simulink model "qcar2LidarToGPS"  (R2023a)
settings: Solver=ode1  StartTime=0.0  StopTime=inf  FixedStep=1/15  RelTol=1e-3  EnableMultiTasking=on
undefined symbols (not defined in the file): Point, qc_get_step_size
libraries: quarc_library x20, simulink x4
settings Model: SimulationMode=external  ExtModeTrigDuration=10000  Creator=PKaram  LastModifiedBy=ZinanCen
settings SolverCC: AlgebraicLoopSolver=TrustRegion  PositivePriorityOrder=on  AutoInsertRateTranBlk=on
settings DataIOCC: ReturnWorkspaceOutputs=off
settings DebuggingCC: ParameterPrecisionLossMsg=none  UnconnectedInputMsg=warning  UnconnectedOutputMsg=warning  UnconnectedLineMsg=warning  ArithmeticOperatorsInVariantConditions=warning
settings HardwareCC: ProdBitPerLong=64  ProdLargestAtomicInteger=LongLong  ProdLargestAtomicFloat=Double  ProdLongLongMode=on  ProdHWDeviceType=ARM Compatible->ARM 64-bit (LP64)
settings ModelReferenceCC: EnableRefExpFcnMdlSchedulingChecks=on
settings SFSimCC: SimUseLocalCustomCode=off  CustomCodeUndefinedFunction=UseInterfaceOnly
settings RTWCC: Description=QUARC Linux QCar2 Target Using Toolchain  SystemTargetFile=quarc_linux_qcar2.tlc  TemplateMakefile=quarc_linux_nvidia_tmf  RTWUseLocalCustomCode=off  Toolchain=QUARC linux_qcar2 | gmake (64-bit Windows)  BuildConfiguration=Faster Runs  DLArmComputeVersion=19.05
settings CodeAppCC: StateflowObjectComments=on
settings STFCustomTargetCC: SystemTargetFile=quarc_linux_qcar2.tlc
settings GRTTargetCC: ParMdlRefBuildCompliant=off  CompOptLevelCompliant=off  CombineOutputUpdateFcns=off  MatFileLogging=off  CPPClassGenCompliant=off  GRTInterface=on  ExtMode=on  ExtModeMexFile=quarc_comm  ExtModeMexArgs='-w -d /home/nvidia/Documents -uri %u -pose_0 [0.],[0.],[0.]','tcpip://192.168.3.38:17001'
settings ConfigComp: CovMetricSettings=dswe

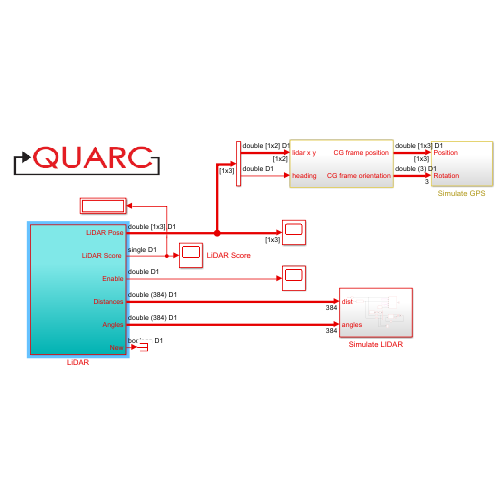
[thumbnail: Simulink's stored preview of the top-level diagram]
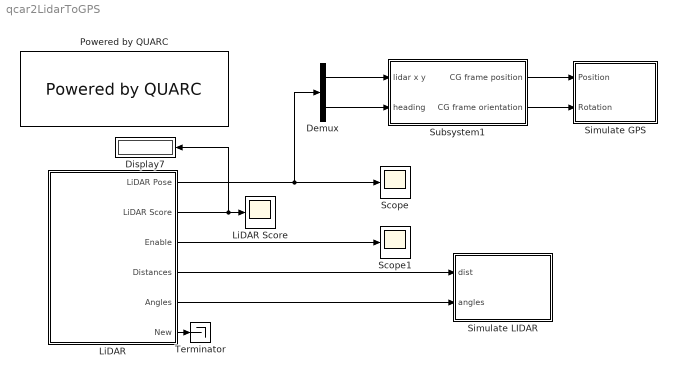
== system qcar2LidarToGPS ==
  Demux : Demux  Outputs=[2 1]
  Display7 : Display
  LiDAR : Subsystem
  LiDAR Score : Scope
  Powered by QUARC : quarc_library/Logos/Powered by QUARC
  Scope : Scope
  Scope1 : Scope
  Simulate GPS : Subsystem
  Simulate LIDAR : Subsystem
  Subsystem1 : Subsystem
  Terminator : Terminator
  wires:
  LiDAR/2("LiDAR Score ") -> Display7/1, LiDAR Score/1
  LiDAR/3(Enable) -> Scope1/1
  LiDAR/1(LiDAR Pose) -> Scope/1, Demux/1
  Demux/1 -> Subsystem1/1(lidar x y)
  Subsystem1/1("CG frame position ") -> Simulate GPS/1(Position)
  Subsystem1/2(CG frame orientation) -> Simulate GPS/2(Rotation)
  Demux/2 -> Subsystem1/2(heading)
  LiDAR/4(Distances) -> Simulate LIDAR/1(dist)
  LiDAR/5(Angles) -> Simulate LIDAR/2(angles)
  LiDAR/6(New) -> Terminator/1

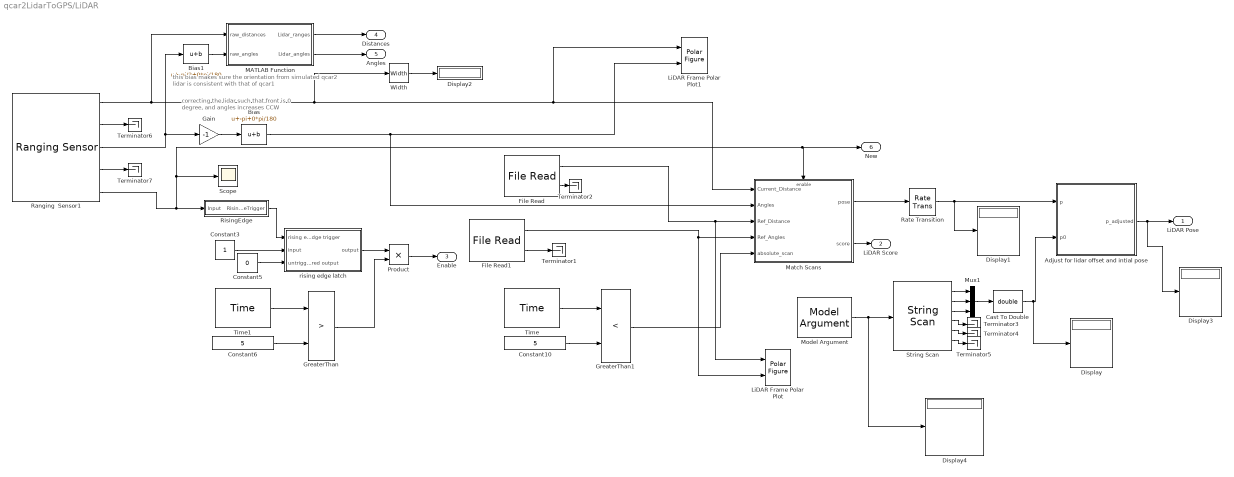
== system qcar2LidarToGPS/LiDAR ==
  note: correcting the lidar such that front is 0 degree, and angles increases CCW
  note: this bias makes sure the orientation from simulated qcar2 lidar is consistent with that of qcar1
  Adjust for lidar offset and intial pose : MATLAB Function  TreatAsAtomicUnit=on
  Bias : Bias  Bias=-pi+0*pi/180  SaturateOnIntegerOverflow=off
  Bias1 : Bias  Bias=-pi/2+0*pi/180  SaturateOnIntegerOverflow=off
  Cast To Double : DataTypeConversion  OutDataTypeStr=double  SaturateOnIntegerOverflow=off  RndMeth=Floor
  Constant10 : Constant  Value=5
  Constant3 : Constant
  Constant5 : Constant  Value=0
  Constant6 : Constant  Value=5
  Display{,1..4} (5 alike) : Display
  File Read : quarc_library/Sources/Signals/File Read  source=Specify via dialog (do not evaluate)  filename=distance_new.mat  format=MAT-file v.4  variable=distances  dimensions=[384, 1]  skip_lines=1  skip_columns=1  loop_count=0  sample_time=qc_get_step_size  data_type=double
      settings: AttributesFormatString="\"distance_new.mat"  SourceProductName=QUARC Targets
  File Read1 : quarc_library/Sources/Signals/File Read  source=Specify via dialog (do not evaluate)  filename=angles_new.mat  format=MAT-file v.4  variable=angles  dimensions=[384, 1]  skip_lines=1  skip_columns=1  loop_count=0  sample_time=qc_get_step_size  data_type=double
      settings: AttributesFormatString="\"angles_new.mat"  SourceProductName=QUARC Targets
  Gain : Gain  Gain=-1
  GreaterThan : RelationalOperator  Operator=>  OutDataTypeStr=boolean  RndMeth=Simplest  InputSameDT=off
  GreaterThan1 : RelationalOperator  Operator=<  OutDataTypeStr=boolean  RndMeth=Simplest  InputSameDT=off
  LiDAR Frame Polar Plot : quarc_library/Sinks/Figures/Polar Figure  figure_mode=Use figure window  figure_tag=figure1  axes_tag=axes1  plot_mode=Frame-based  minimum_rho=0  maximum_rho=5  minimum_theta=0  maximum_theta=360  zero_location=top  direction=counterclockwise  buffer_size=1  update_rate=1  sample_time=-1  initial_position="1541.8           49.8          766.4          758.4"  initial_visibility=off  line1_style=None  line1_width=1  line1_color=[0 0 0]  marker1=Point (.)  marker1_size=1  marker1_edge_color=[0 0.447059 0.741176]  marker1_face_color=[0 0.447059 0.741176]  line2_style=Solid line (-)  line2_width=0.5  line2_color=[0.85098 0.32549 0.0980392]  marker2=None  marker2_size=6  marker2_edge_color=[0.85098 0.32549 0.0980392]  marker2_face_color=[0.85098 0.32549 0.0980392]  line3_style=Solid line (-)  line3_width=0.5  line3_color=[0.929412 0.694118 0.12549]  marker3=None  marker3_size=6  marker3_edge_color=[0.929412 0.694118 0.12549]  marker3_face_color=[0.929412 0.694118 0.12549]  line4_style=Solid line (-)  line4_width=0.5  line4_color=[0.494118 0.184314 0.556863]  marker4=None  marker4_size=6  marker4_edge_color=[0.494118 0.184314 0.556863]  marker4_face_color=[0.494118 0.184314 0.556863]  line5_style=Solid line (-)  line5_width=0.5  line5_color=[0.466667 0.67451 0.188235]  marker5=None  marker5_size=6  marker5_edge_color=[0.466667 0.67451 0.188235]  marker5_face_color=[0.466667 0.67451 0.188235]
      settings: SourceProductName=QUARC Targets
  LiDAR Frame Polar Plot1 : quarc_library/Sinks/Figures/Polar Figure  figure_mode=Use figure window  figure_tag=figure1  axes_tag=axes1  plot_mode=Frame-based  minimum_rho=0  maximum_rho=5  minimum_theta=0  maximum_theta=360  zero_location=top  direction=counterclockwise  buffer_size=1  update_rate=1  sample_time=-1  initial_position="2305.8           49.8          766.4          758.4"  initial_visibility=off  line1_style=None  line1_width=1  line1_color=[0 0 0]  marker1=Point (.)  marker1_size=1  marker1_edge_color=[0 0.447059 0.741176]  marker1_face_color=[0 0.447059 0.741176]  line2_style=Solid line (-)  line2_width=0.5  line2_color=[0.85098 0.32549 0.0980392]  marker2=None  marker2_size=6  marker2_edge_color=[0.85098 0.32549 0.0980392]  marker2_face_color=[0.85098 0.32549 0.0980392]  line3_style=Solid line (-)  line3_width=0.5  line3_color=[0.929412 0.694118 0.12549]  marker3=None  marker3_size=6  marker3_edge_color=[0.929412 0.694118 0.12549]  marker3_face_color=[0.929412 0.694118 0.12549]  line4_style=Solid line (-)  line4_width=0.5  line4_color=[0.494118 0.184314 0.556863]  marker4=None  marker4_size=6  marker4_edge_color=[0.494118 0.184314 0.556863]  marker4_face_color=[0.494118 0.184314 0.556863]  line5_style=Solid line (-)  line5_width=0.5  line5_color=[0.466667 0.67451 0.188235]  marker5=None  marker5_size=6  marker5_edge_color=[0.466667 0.67451 0.188235]  marker5_face_color=[0.466667 0.67451 0.188235]
      settings: SourceProductName=QUARC Targets
  MATLAB Function : MATLAB Function  TreatAsAtomicUnit=on
  Match Scans : Subsystem
  Model Argument : quarc_library/Sources/Signals/Model Argument  argument_name=pose_0  has_value=on  data_type_mode=Specify via dialog  data_type=char  max_length=80  default_value=0  default_string=0,0,0  variable_size=on
      settings: AttributesFormatString=(-%<argument_name>)  SourceProductName=QUARC Targets
  Mux1 : Mux  Inputs=3
  Product : Product
  Ranging  Sensor1 : quarc_library/Devices/Third-Party/Sensors/Ranging Sensor  sensor_type=RPLidar LIDAR  uri=serial-cpu://localhost:1?baud='256000',word='8',parity='none',stop='1',flow='none',dsr='on'  ranging_distance=Long  timing_budget=0.033  measurement_period=0.0005  output_mode=Fixed-size interpolated output  samples_per_revolution=384  max_distance=0.050  max_angle=5  sample_time=qc_get_step_size  show_versions=off  active=on
      settings: SourceProductName=QUARC Targets
  Rate Transition : RateTransition
  RisingEdge : Subsystem
  Scope : Scope
  String Scan : quarc_library/Strings/String Scan  format_string=%e, %f, %g  max_length=80
      settings: SourceProductName=QUARC Targets
  Terminator{1..7} (7 alike) : Terminator
  Time : quarc_library/Sources/Time/Time  time_source=Wall clock  sample_time=qc_get_step_size
  Time1 : quarc_library/Sources/Time/Time  time_source=Wall clock  sample_time=qc_get_step_size
  Width : Width
  rising edge latch : Subsystem
  LiDAR Pose : Outport
  "LiDAR Score " : Outport  Port=2
  Enable : Outport  Port=3
  Distances : Outport  Port=4
  Angles : Outport  Port=5
  New : Outport  Port=6
  wires:
  File Read/1 -> LiDAR Frame Polar Plot/1, Match Scans/3(Ref_Distance)
  Width/1 -> Display2/1
  Ranging  Sensor1/1 -> MATLAB Function/1(raw_distances), Width/1, LiDAR Frame Polar Plot1/1, Match Scans/1(Current_Distance)
  Match Scans/1(pose) -> Rate Transition/1
  Constant6/1 -> GreaterThan/2
  RisingEdge/1(RisingEdgeTrigger) -> rising edge latch/1(rising edge trigger)
  Match Scans/2(score) -> "LiDAR Score "/1
  Product/1 -> Enable/1
  Constant3/1 -> rising edge latch/2(input)
  Constant5/1 -> rising edge latch/3(untriggered output)
  Constant10/1 -> GreaterThan1/2
  GreaterThan/1 -> Product/2
  Time/1 -> GreaterThan1/1
  GreaterThan1/1 -> Match Scans/5(absolute_scan)
  Time1/1 -> GreaterThan/1
  rising edge latch/1(output) -> Product/1
  Bias/1 -> Match Scans/2(Angles), LiDAR Frame Polar Plot1/2
  Ranging  Sensor1/5 -> New/1, Match Scans/Enable, Scope/1, RisingEdge/1(Input)
  File Read1/1 -> LiDAR Frame Polar Plot/2, Match Scans/4(Ref_Angles)
  File Read1/2 -> Terminator1/1
  File Read/2 -> Terminator2/1
  Model Argument/1 -> Display4/1, String Scan/1
  String Scan/4 -> Terminator3/1
  String Scan/5 -> Terminator4/1
  String Scan/6 -> Terminator5/1
  MATLAB Function/1(Lidar_ranges) -> Distances/1
  MATLAB Function/2(Lidar_angles) -> Angles/1
  Mux1/1 -> Cast To Double/1
  String Scan/1 -> Mux1/1
  String Scan/2 -> Mux1/2
  String Scan/3 -> Mux1/3
  Adjust for lidar offset and intial pose/1(p_adjusted) -> Display3/1, LiDAR Pose/1
  Rate Transition/1 -> Display1/1, Adjust for lidar offset and intial pose/1(p)
  Cast To Double/1 -> Display/1, Adjust for lidar offset and intial pose/2(p0)
  Ranging  Sensor1/2 -> Terminator6/1
  Ranging  Sensor1/4 -> Terminator7/1
  Gain/1 -> Bias/1
  Ranging  Sensor1/3 -> Bias1/1, Gain/1
  Bias1/1 -> MATLAB Function/2(raw_angles)

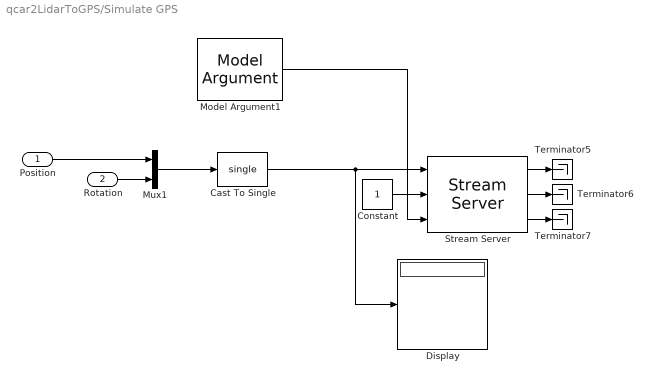
== system qcar2LidarToGPS/Simulate GPS ==
  Position : Inport
  Rotation : Inport  Port=2
  Cast To Single : DataTypeConversion  OutDataTypeStr=single  SaturateOnIntegerOverflow=off  RndMeth=Floor
  Constant : Constant
  Display : Display
  Model Argument1 : quarc_library/Sources/Signals/Model Argument  argument_name=uri_gps  has_value=on  data_type_mode=Specify via dialog  data_type=char  max_length=80  default_value=0  default_string=tcpip://remotehost:18967  variable_size=off
      settings: AttributesFormatString=(-%<argument_name>)  SourceProductName=QUARC Targets
  Mux1 : Mux  Inputs=2
  Stream Server : quarc_library/Communications/Basic/Stream Server  uri_source=External input port  uri=tcpip://remotehost:18967  send_buffer_size=1460  receive_buffer_size=1460  byte_order=little endian (Intel - LSB first)  optimization=Minimum latency  send_options=Send most recent data  receive_options=Do not receive data  default_value=[0]  sample_time=qc_get_step_size*3  active=off  implementation=Use blocking I/O in a separate thread  send_fifo_size=1000  receive_fifo_size=1000  send_priority=0  receive_priority=0  send_dimensions=off  receive_dimensions=off  max_dimensions=-1  data_type=Inherited via back propagation  type_expr=BusObject
  Terminator5 : Terminator
  Terminator6 : Terminator
  Terminator7 : Terminator
  wires:
  Rotation/1 -> Mux1/2
  Stream Server/1 -> Terminator5/1
  Stream Server/2 -> Terminator6/1
  Stream Server/3 -> Terminator7/1
  Constant/1 -> Stream Server/2
  Position/1 -> Mux1/1
  Mux1/1 -> Cast To Single/1
  Cast To Single/1 -> Display/1, Stream Server/1
  Model Argument1/1 -> Stream Server/3

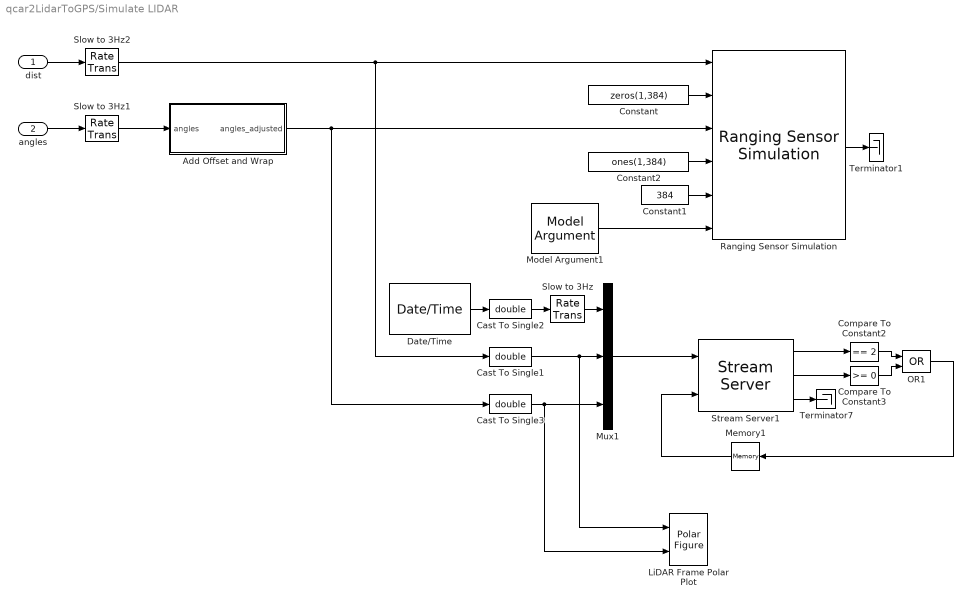
== system qcar2LidarToGPS/Simulate LIDAR ==
  dist : Inport
  angles : Inport  Port=2
  Add Offset and Wrap : MATLAB Function  TreatAsAtomicUnit=on
  Cast To Single1 : DataTypeConversion  OutDataTypeStr=double  SaturateOnIntegerOverflow=off  RndMeth=Floor
  Cast To Single2 : DataTypeConversion  OutDataTypeStr=double  SaturateOnIntegerOverflow=off  RndMeth=Floor
  Cast To Single3 : DataTypeConversion  OutDataTypeStr=double  SaturateOnIntegerOverflow=off  RndMeth=Floor
  Compare To Constant2 : simulink/Logic and Bit Operations/Compare To Constant  relop===  const=2  OutDataTypeStr=boolean
  Compare To Constant3 : simulink/Logic and Bit Operations/Compare To Constant  relop=>=  const=0  OutDataTypeStr=boolean
  Constant : Constant  Value=zeros(1,384)
  Constant1 : Constant  Value=384
  Constant2 : Constant  Value=ones(1,384)
  Date/Time : quarc_library/Sources/Time/Date//Time  show_date=off  show_time=off  show_epoch=on  use_utc=off  sample_time=-1
      settings: SourceProductName=QUARC Targets
  LiDAR Frame Polar Plot : quarc_library/Sinks/Figures/Polar Figure  figure_mode=Use figure window  figure_tag=figure1  axes_tag=axes1  plot_mode=Frame-based  minimum_rho=0  maximum_rho=5  minimum_theta=0  maximum_theta=360  zero_location=top  direction=counterclockwise  buffer_size=1  update_rate=1  sample_time=-1  initial_position="2306.3333      50.333333      765.33333      758.66667"  initial_visibility=off  line1_style=None  line1_width=1  line1_color=[0 0 0]  marker1=Point (.)  marker1_size=1  marker1_edge_color=[0 0.447059 0.741176]  marker1_face_color=[0 0.447059 0.741176]  line2_style=Solid line (-)  line2_width=0.5  line2_color=[0.85098 0.32549 0.0980392]  marker2=None  marker2_size=6  marker2_edge_color=[0.85098 0.32549 0.0980392]  marker2_face_color=[0.85098 0.32549 0.0980392]  line3_style=Solid line (-)  line3_width=0.5  line3_color=[0.929412 0.694118 0.12549]  marker3=None  marker3_size=6  marker3_edge_color=[0.929412 0.694118 0.12549]  marker3_face_color=[0.929412 0.694118 0.12549]  line4_style=Solid line (-)  line4_width=0.5  line4_color=[0.494118 0.184314 0.556863]  marker4=None  marker4_size=6  marker4_edge_color=[0.494118 0.184314 0.556863]  marker4_face_color=[0.494118 0.184314 0.556863]  line5_style=Solid line (-)  line5_width=0.5  line5_color=[0.466667 0.67451 0.188235]  marker5=None  marker5_size=6  marker5_edge_color=[0.466667 0.67451 0.188235]  marker5_face_color=[0.466667 0.67451 0.188235]
      settings: SourceProductName=QUARC Targets
  Memory1 : Memory  InheritSampleTime=on
  Model Argument1 : quarc_library/Sources/Signals/Model Argument  argument_name=uri_lidar  has_value=on  data_type_mode=Specify via dialog  data_type=char  max_length=80  default_value=0  default_string=tcpip://localhost:18966  variable_size=off
      settings: AttributesFormatString=(-%<argument_name>)  SourceProductName=QUARC Targets
  Mux1 : Mux  Inputs=3
  OR1 : Logic  Operator=OR  IconShape=distinctive  AllPortsSameDT=off  OutDataTypeStr=boolean
  Ranging Sensor Simulation : quarc_library/Devices/Third-Party/Sensors/Ranging Sensor Simulation  sensor_type=RPLIDAR A2  uri_source=External input port  uri=tcpip://localhost:18966  sample_time=qc_get_step_size  show_in_use=off  variable_size=off  active=on
      settings: SourceProductName=QUARC Targets
  Slow to 3Hz : RateTransition  OutPortSampleTime=qc_get_step_size*ceil(1/15 / qc_get_step_size)
  Slow to 3Hz1 : RateTransition  OutPortSampleTime=qc_get_step_size*ceil(1/15 / qc_get_step_size)
  Slow to 3Hz2 : RateTransition  OutPortSampleTime=qc_get_step_size*ceil(1/15 / qc_get_step_size)
  Stream Server1 : quarc_library/Communications/Basic/Stream Server  uri_source=Specify via dialog (do not evaluate)  uri=tcpip://localhost:18968  send_buffer_size=8*(384*2 +1)  receive_buffer_size=1  byte_order=little endian (Intel - LSB first)  optimization=Minimum latency  send_options=Send most recent data  receive_options=Do not receive data  default_value=[0]  sample_time=qc_get_step_size*ceil(1/15 / qc_get_step_size)  active=off  implementation=Use non-blocking I/O  send_fifo_size=1  receive_fifo_size=1000  send_priority=0  receive_priority=0  send_dimensions=off  receive_dimensions=off  max_dimensions=-1  data_type=Inherited via back propagation  type_expr=BusObject
      settings: AttributesFormatString="\"tcpip://localhost:18968\""
  Terminator1 : Terminator
  Terminator7 : Terminator
  wires:
  Constant/1 -> Ranging Sensor Simulation/2
  Constant1/1 -> Ranging Sensor Simulation/5
  Constant2/1 -> Ranging Sensor Simulation/4
  Ranging Sensor Simulation/1 -> Terminator1/1
  dist/1 -> Slow to 3Hz2/1
  Model Argument1/1 -> Ranging Sensor Simulation/6
  Mux1/1 -> Stream Server1/1
  Compare To Constant3/1 -> OR1/2
  angles/1 -> Slow to 3Hz1/1
  Slow to 3Hz/1 -> Mux1/1
  Stream Server1/3 -> Terminator7/1
  Compare To Constant2/1 -> OR1/1
  OR1/1 -> Memory1/1
  Stream Server1/2 -> Compare To Constant3/1
  Stream Server1/1 -> Compare To Constant2/1
  Cast To Single3/1 -> LiDAR Frame Polar Plot/2, Mux1/3
  Cast To Single2/1 -> Slow to 3Hz/1
  Date/Time/1 -> Cast To Single2/1
  Cast To Single1/1 -> LiDAR Frame Polar Plot/1, Mux1/2
  Memory1/1 -> Stream Server1/2
  Slow to 3Hz2/1 -> Ranging Sensor Simulation/1, Cast To Single1/1
  Slow to 3Hz1/1 -> Add Offset and Wrap/1(angles)
  Add Offset and Wrap/1(angles_adjusted) -> Ranging Sensor Simulation/3, Cast To Single3/1

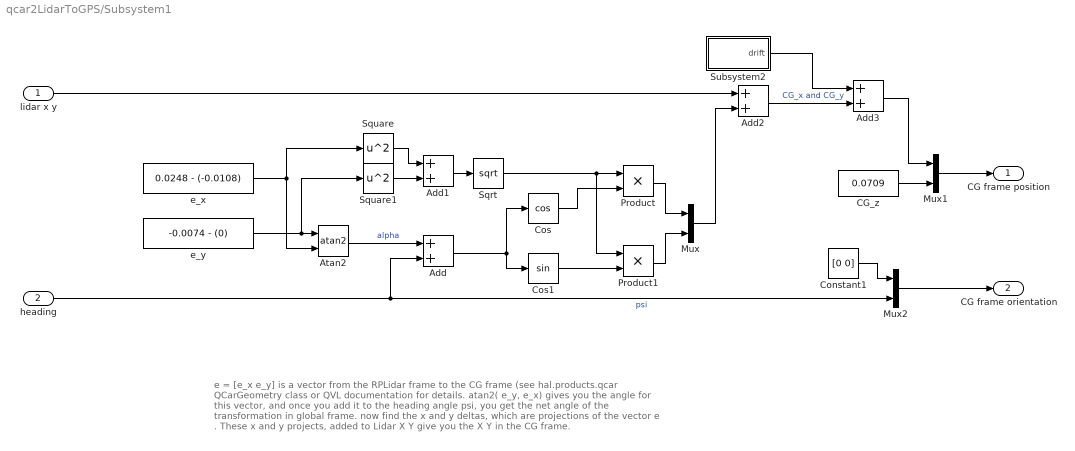
== system qcar2LidarToGPS/Subsystem1 ==
  note: e = [e_x e_y] is a vector from the RPLidar frame to the CG frame (see hal.products.qcar QCarGeometry class or QVL documentation for details.
      |
      | atan2( e_y, e_x) gives you the angle for this vector, and once you add it to the heading angle psi, you get the net angle of the transformation in global frame. now find the x and y deltas, which are projections of the vector e . These x and y projects, added to Lidar X Y give you the X Y in the CG frame.
  lidar x y : Inport
  heading : Inport  Port=2
  Add{,1..3} (4 alike) : Sum
  Atan2 : Trigonometry  Operator=atan2
  CG_z : Constant  Value=0.0709
  Constant1 : Constant  Value=[0 0]
  Cos : Trigonometry  Operator=cos
  Cos1 : Trigonometry
  Mux : Mux  Inputs=2
  Mux1 : Mux  Inputs=2
  Mux2 : Mux  Inputs=2
  Product : Product
  Product1 : Product
  Sqrt : Sqrt
  Square : Math  Operator=square
  Square1 : Math  Operator=square
  Subsystem2 : Subsystem
  e_x : Constant  Value=0.0248 - (-0.0108)
  e_y : Constant  Value=-0.0074 - (0)
  "CG frame position " : Outport
  CG frame orientation : Outport  Port=2
  wires:
  e_y/1 -> Square1/1, Atan2/1
  e_x/1 -> Square/1, Atan2/2
  Atan2/1 -> Add/1  "alpha"
  heading/1 -> Mux2/2, Add/2  "psi"
  Square/1 -> Add1/1
  Square1/1 -> Add1/2
  Add1/1 -> Sqrt/1
  Add/1 -> Cos1/1, Cos/1
  Sqrt/1 -> Product1/1, Product/1
  Cos/1 -> Product/2
  Cos1/1 -> Product1/2
  Product/1 -> Mux/1
  Product1/1 -> Mux/2
  Mux/1 -> Add2/2
  lidar x y/1 -> Add2/1
  Add2/1 -> Add3/2  "CG_x and CG_y"
  CG_z/1 -> Mux1/2
  Constant1/1 -> Mux2/1
  Mux1/1 -> "CG frame position "/1
  Mux2/1 -> CG frame orientation/1
  Subsystem2/1(drift) -> Add3/1
  Add3/1 -> Mux1/1

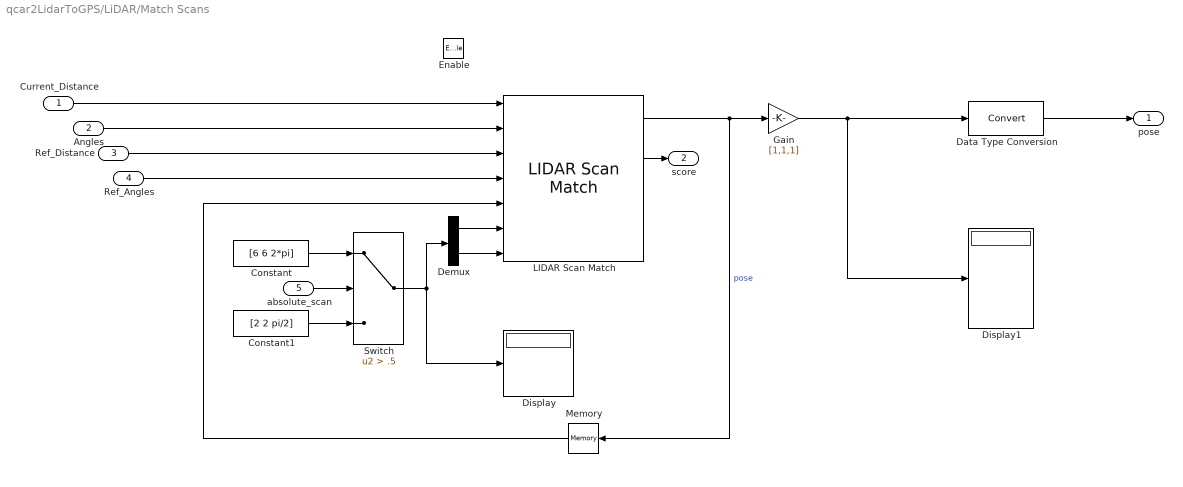
== system qcar2LidarToGPS/LiDAR/Match Scans ==
  Current_Distance : Inport
  Angles : Inport  Port=2
  Ref_Distance : Inport  Port=3
  Ref_Angles : Inport  Port=4
  absolute_scan : Inport  Port=5
  Enable : EnablePort
  Constant : Constant  Value=[6 6 2*pi]
  Constant1 : Constant  Value=[2 2 pi/2]
  Data Type Conversion : DataTypeConversion  SaturateOnIntegerOverflow=off  RndMeth=Floor
  Demux : Demux  Outputs=2
  Display : Display
  Display1 : Display
  Gain : Gain  Gain=[1,1,1]
  LIDAR Scan Match : quarc_library/Image Processing/Generic/LIDAR Scan Match  mode=Variable-size input  resolution=30  max_range=6  use_initial_pose=on
      settings: SourceProductName=QUARC Targets
  Memory : Memory  InitialCondition=[0 0 0]  InheritSampleTime=on  LinearizeMemory=on  LinearizeAsDelay=on
  Switch : Switch  Criteria=u2 > Threshold  Threshold=.5  SaturateOnIntegerOverflow=off  InputSameDT=off
  pose : Outport
  score : Outport  Port=2
  wires:
  LIDAR Scan Match/1 -> Gain/1, Memory/1  "pose"
  Current_Distance/1 -> LIDAR Scan Match/1
  Ref_Distance/1 -> LIDAR Scan Match/3
  Angles/1 -> LIDAR Scan Match/2
  Ref_Angles/1 -> LIDAR Scan Match/4
  LIDAR Scan Match/2 -> score/1
  Memory/1 -> LIDAR Scan Match/5
  absolute_scan/1 -> Switch/2
  Switch/1 -> Demux/1, Display/1
  Demux/1 -> LIDAR Scan Match/6
  Demux/2 -> LIDAR Scan Match/7
  Constant/1 -> Switch/1
  Constant1/1 -> Switch/3
  Data Type Conversion/1 -> pose/1
  Gain/1 -> Data Type Conversion/1, Display1/1

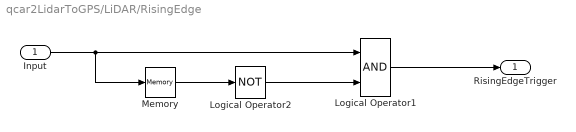
== system qcar2LidarToGPS/LiDAR/RisingEdge ==
  Input : Inport
  Logical Operator1 : Logic  AllPortsSameDT=off
  Logical Operator2 : Logic  Operator=NOT  AllPortsSameDT=off
  Memory : Memory  InheritSampleTime=on  LinearizeMemory=on
  RisingEdgeTrigger : Outport  VectorParamsAs1DForOutWhenUnconnected=off
  wires:
  Logical Operator1/1 -> RisingEdgeTrigger/1
  Logical Operator2/1 -> Logical Operator1/2
  Memory/1 -> Logical Operator2/1
  Input/1 -> Logical Operator1/1, Memory/1

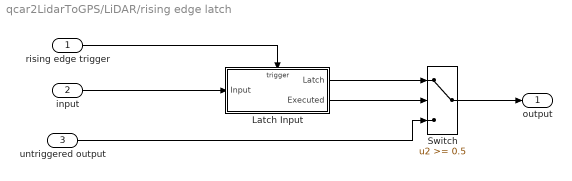
== system qcar2LidarToGPS/LiDAR/rising edge latch ==
  rising edge trigger : Inport
  input : Inport  Port=2
  untriggered output : Inport  Port=3
  Latch Input : Subsystem  TreatAsAtomicUnit=on
  Switch : Switch  Threshold=0.5  SaturateOnIntegerOverflow=off  InputSameDT=off
  output : Outport  VectorParamsAs1DForOutWhenUnconnected=off
  wires:
  untriggered output/1 -> Switch/3
  Switch/1 -> output/1
  Latch Input/1(Latch) -> Switch/1
  Latch Input/2(Executed) -> Switch/2
  input/1 -> Latch Input/1(Input)
  rising edge trigger/1 -> Latch Input/Trigger

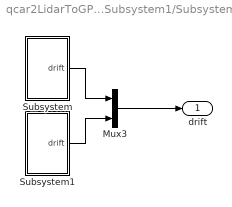
== system qcar2LidarToGPS/Subsystem1/Subsystem2 ==
  Mux3 : Mux  Inputs=2
  Subsystem : Subsystem
  Subsystem1 : Subsystem
  drift : Outport
  wires:
  Subsystem1/1(drift) -> Mux3/2
  Subsystem/1(drift) -> Mux3/1
  Mux3/1 -> drift/1

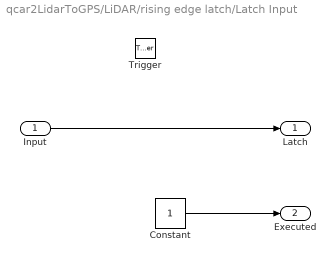
== system qcar2LidarToGPS/LiDAR/rising edge latch/Latch Input ==
  Input : Inport
  Trigger : TriggerPort  VariantControl=(inherit)
  Constant : Constant
  Latch : Outport  VectorParamsAs1DForOutWhenUnconnected=off
  Executed : Outport  Port=2  VectorParamsAs1DForOutWhenUnconnected=off
  wires:
  Constant/1 -> Executed/1
  Input/1 -> Latch/1

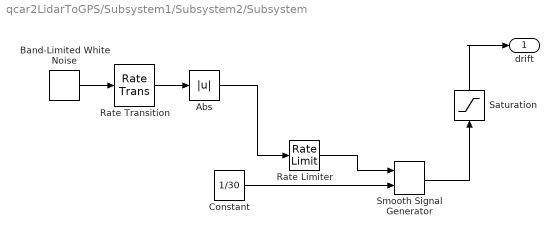
== system qcar2LidarToGPS/Subsystem1/Subsystem2/Subsystem ==
  Abs : Abs  SaturateOnIntegerOverflow=off
  Band-Limited White Noise : simulink/Sources/Band-Limited White Noise  Cov=[0.002]  Ts=5  seed=randi(23341)
  Constant : Constant  Value=1/30  SampleTime=1/15
  Rate Limiter : RateLimiter  RisingSlewLimit=0.1  SampleTimeMode=inherited
  Rate Transition : RateTransition
  Saturation : Saturate  UpperLimit=0.07/sqrt(2)  LowerLimit=-0.07/sqrt(2)
  Smooth Signal Generator : quarc_library/Sources/Signals/Smooth Signal Generator  signal_type=Sine  source=External (input ports)  amplitude=1  frequency=1  initial_phase=randi(360)*pi/180  sample_time=qc_get_step_size  output_cos=off
      settings: SourceProductName=QUARC Targets
  drift : Outport
  wires:
  Band-Limited White Noise/1 -> Rate Transition/1
  Smooth Signal Generator/1 -> Saturation/1
  Abs/1 -> Rate Limiter/1
  Rate Limiter/1 -> Smooth Signal Generator/1
  Rate Transition/1 -> Abs/1
  Constant/1 -> Smooth Signal Generator/2
  Saturation/1 -> drift/1

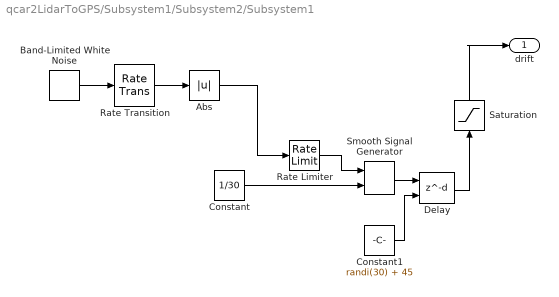
== system qcar2LidarToGPS/Subsystem1/Subsystem2/Subsystem1 ==
  Abs : Abs  SaturateOnIntegerOverflow=off
  Band-Limited White Noise : simulink/Sources/Band-Limited White Noise  Cov=[0.002]  Ts=5  seed=randi(23341)
  Constant : Constant  Value=1/30  SampleTime=1/15
  Constant1 : Constant  Value=randi(30) + 45
  Delay : Delay  DelayLengthSource=Input port  DelayLength=randi(30) + 45
      settings: InputPortMap=u0,p1
  Rate Limiter : RateLimiter  RisingSlewLimit=0.1  SampleTimeMode=inherited
  Rate Transition : RateTransition
  Saturation : Saturate  UpperLimit=0.07/sqrt(2)  LowerLimit=-0.07/sqrt(2)
  Smooth Signal Generator : quarc_library/Sources/Signals/Smooth Signal Generator  signal_type=Sine  source=External (input ports)  amplitude=1  frequency=1  initial_phase=randi(360)*pi/180  sample_time=qc_get_step_size  output_cos=off
      settings: SourceProductName=QUARC Targets
  drift : Outport
  wires:
  Constant/1 -> Smooth Signal Generator/2
  Rate Transition/1 -> Abs/1
  Rate Limiter/1 -> Smooth Signal Generator/1
  Abs/1 -> Rate Limiter/1
  Smooth Signal Generator/1 -> Delay/1
  Band-Limited White Noise/1 -> Rate Transition/1
  Saturation/1 -> drift/1
  Delay/1 -> Saturation/1
  Constant1/1 -> Delay/2

== matlab function qcar2LidarToGPS/LiDAR/MATLAB Function ==
  data: raw_distances input size=384; Lidar_ranges output; raw_angles input size=384; Lidar_angles output
function [Lidar_ranges,Lidar_angles]= fcn(raw_distances, raw_angles)

%  Fixed sized vector used for streaming the LiDAR values 
Lidar_ranges = zeros(384,1);
Lidar_angles = zeros(384,1);


Lidar_ranges(:)  = raw_distances;
Lidar_angles(:) =  raw_angles;

== matlab function qcar2LidarToGPS/Simulate LIDAR/Add Offset and Wrap ==
  data: angles input size=384; angles_adjusted output size=384
function angles_adjusted = fcn(angles)


angles_adjusted = wrapTo2Pi(angles + 3*pi/2);

== matlab function qcar2LidarToGPS/LiDAR/Adjust for lidar offset and intial pose ==
  data: p input; p_adjusted output; p0 input
function p_adjusted = fcn(p, p0)

x0 = p0(1);
y0 = p0(2);
th0 = p0(3);

x = p(1);
y = p(2);
th = p(3);

x_adj = x0 + x*cos(th0) - y*sin(th0);
y_adj = y0 + x*sin(th0) + y*cos(th0);
th_adj = wrapToPi(th0 + th);

p_adjusted = [x_adj, y_adj, th_adj];
